simulink model "Simplified_Wind_Turbine_model"  (R2023b)
settings: Solver=ode23t  StartTime=0.0  StopTime=simT  RelTol=1e-3  AbsTol=1e-3
PreLoadFcn:
  | sscv_wind_turbine_input
values from neighbouring files (symbols this model uses):
  actuatorRampRate = 20    [sscv_wind_turbine_input.m]
  brakePressure = 100    [sscv_wind_turbine_input.m]
  controllerTimeConstant = 2    [sscv_wind_turbine_input.m]
  cumulativeStressThreshold = 1.5e6    (= 1500000)    [sscv_wind_turbine_input.m]
  generatorEfficiency = 90    [sscv_wind_turbine_input.m]
  iGenerationGain = 1    [sscv_wind_turbine_input.m]
  initialOperationTime = 0    [sscv_wind_turbine_input.m]
  inizialStressThreshold = 500e3    (= 500000)    [sscv_wind_turbine_input.m]
  maxPitchAngle = max(pitch)    [sscv_wind_turbine_input.m]
  minPitchAngle = min(pitch)    [sscv_wind_turbine_input.m]
  pGenerationGain = 0.1    [sscv_wind_turbine_input.m]
  pGeneratorBrakeLimit = 0.50    (= 0.5)    [sscv_wind_turbine_input.m]
  pitchBrakeAngle = 95    [sscv_wind_turbine_input.m]
  stressRateRelease = 0.05    [sscv_wind_turbine_input.m]
  transformerRatedPower = 1.8    [sscv_wind_turbine_input.m]
  turbineRatedPower = 1.5    [sscv_wind_turbine_input.m]
  vWindRated = 12    [sscv_wind_turbine_input.m]
  wAtGeneratorRatedPower = wTurbineCutOut*gearRatio    (= 1227.93)    [sscv_wind_turbine_input.m]
  wearRate = 0.033    [sscv_wind_turbine_input.m]
  wGeneratorBrakeLimit = 0.50    (= 0.5)    [sscv_wind_turbine_input.m]
  wTurbineCutOut = 22    [sscv_wind_turbine_input.m]
undefined symbols (not defined in the file or in its folder): Derating, mpptOmega, mpptPower, mpptWindSpeed
libraries: fl_lib x22, simulink x14, nesl_utility x11, sdl_lib x10, dspnetwork x3, simulink_extras x3
(part 2 of 2)

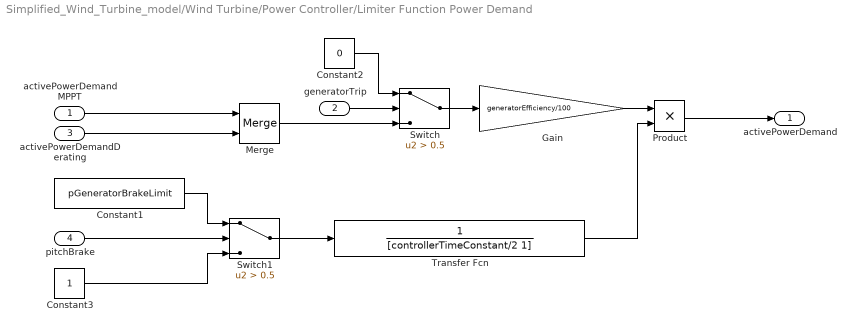
== system Simplified_Wind_Turbine_model/Wind Turbine/Power Controller/Limiter Function Power Demand ==
  activePowerDemandMPPT : Inport
  generatorTrip : Inport  Port=2
  activePowerDemandDerating : Inport  Port=3
  pitchBrake : Inport  Port=4
  Constant1 : Constant  Value=pGeneratorBrakeLimit
  Constant2 : Constant  Value=0
  Constant3 : Constant
  Gain : Gain  Gain=generatorEfficiency/100
  Merge : Merge
  Product : Product
  Switch : Switch  Criteria=u2 > Threshold  Threshold=0.5  SaturateOnIntegerOverflow=off  InputSameDT=off
  Switch1 : Switch  Criteria=u2 > Threshold  Threshold=0.5  SaturateOnIntegerOverflow=off  InputSameDT=off
  Transfer Fcn : TransferFcn  Denominator=[controllerTimeConstant/2 1]
  activePowerDemand : Outport
  wires:
  generatorTrip/1 -> Switch/2
  Switch/1 -> Gain/1
  Constant2/1 -> Switch/1
  Merge/1 -> Switch/3
  activePowerDemandMPPT/1 -> Merge/1
  activePowerDemandDerating/1 -> Merge/2
  pitchBrake/1 -> Switch1/2
  Constant3/1 -> Switch1/3
  Constant1/1 -> Switch1/1
  Gain/1 -> Product/1
  Switch1/1 -> Transfer Fcn/1
  Product/1 -> activePowerDemand/1
  Transfer Fcn/1 -> Product/2

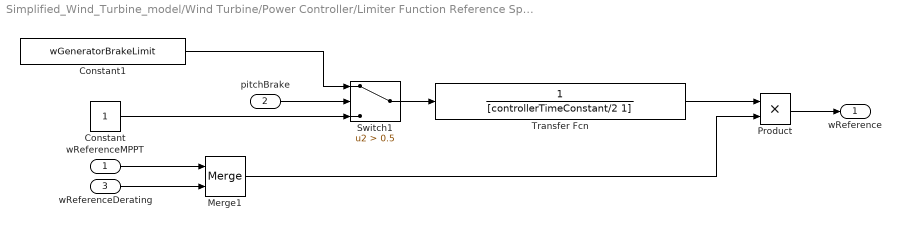
== system Simplified_Wind_Turbine_model/Wind Turbine/Power Controller/Limiter Function Reference Speed ==
  wReferenceMPPT : Inport
  pitchBrake : Inport  Port=2
  wReferenceDerating : Inport  Port=3
  Constant : Constant
  Constant1 : Constant  Value=wGeneratorBrakeLimit
  Merge1 : Merge
  Product : Product
  Switch1 : Switch  Criteria=u2 > Threshold  Threshold=0.5  SaturateOnIntegerOverflow=off  InputSameDT=off
  Transfer Fcn : TransferFcn  Denominator=[controllerTimeConstant/2 1]
  wReference : Outport
  wires:
  pitchBrake/1 -> Switch1/2
  Constant1/1 -> Switch1/1
  wReferenceMPPT/1 -> Merge1/1
  wReferenceDerating/1 -> Merge1/2
  Merge1/1 -> Product/2
  Constant/1 -> Switch1/3
  Product/1 -> wReference/1
  Transfer Fcn/1 -> Product/1
  Switch1/1 -> Transfer Fcn/1

== system Simplified_Wind_Turbine_model/Wind Turbine/Power Controller/MPPT Control ==
  windSpeed : Inport
  Enable : EnablePort  StatesWhenEnabling=reset
  MW to W : Gain  Gain=1e6
  mpptActivePowerDemand : Lookup_n-D  NumberOfTableDimensions=1  BreakpointsForDimension1=mpptWindSpeed  BeginIndexSearchUsingPreviousIndexResult=on  Table=mpptPower  InternalRulePriority=Speed  RndMeth=Simplest
  mpptOmega : Lookup_n-D  NumberOfTableDimensions=1  BreakpointsForDimension1=mpptWindSpeed  BeginIndexSearchUsingPreviousIndexResult=on  Table=mpptOmega  InternalRulePriority=Speed  RndMeth=Simplest
  wReference : Outport
  activePowerDemand : Outport  Port=2
  wires:
  mpptActivePowerDemand/1 -> MW to W/1
  mpptOmega/1 -> wReference/1
  windSpeed/1 -> mpptActivePowerDemand/1, mpptOmega/1
  MW to W/1 -> activePowerDemand/1

== system Simplified_Wind_Turbine_model/Wind Turbine/Gear Tain/Overstress Detector/FaultSystem ==
  Stress : Inport
  StressThreshold : Inport  Port=2
  Compare To Constant : simulink/Logic and Bit Operations/Compare To Constant  relop=>  const=cumulativeStressThreshold  OutDataTypeStr=boolean
  Gain : Gain  Gain=-1*stressRateRelease
  Integrator : Integrator
  Relational Operator : RelationalOperator  Operator=>  OutDataTypeStr=boolean  RndMeth=Simplest  InputSameDT=off
  Switch : Switch  Criteria=u2 > Threshold  SaturateOnIntegerOverflow=off  InputSameDT=off
  fault : Outport
  wires:
  Relational Operator/1 -> Switch/2
  Gain/1 -> Switch/3
  Switch/1 -> Integrator/1
  Integrator/1 -> Compare To Constant/1, Gain/1  "Cumulative Stress"
  StressThreshold/1 -> Relational Operator/2
  Compare To Constant/1 -> fault/1
  Stress/1 -> Switch/1, Relational Operator/1

== system Simplified_Wind_Turbine_model/Wind Turbine/Gear Tain/Overstress Detector/Wear ==
  Bias : Bias  Bias=initialOperationTime  SaturateOnIntegerOverflow=off
  Constant1 : Constant  Value=1/(365*24*60*60)
  Gain1 : Gain  Gain=-1*wearRate
  Integrator1 : Integrator
  Math Function : Math
  Out1 : Outport
  wires:
  Gain1/1 -> Math Function/1
  Constant1/1 -> Integrator1/1
  Math Function/1 -> Out1/1
  Integrator1/1 -> Bias/1
  Bias/1 -> Gain1/1

== stateflow chart Simplified_Wind_Turbine_model/Turbine State Machine ==
  state Startup
    entry: parkingBrake = 0;
    generatorTrip = 1;
    pitchBrake = 0;
    turbineState = 1;
  state Generating
    entry: parkingBrake = 0;
    generatorTrip = 0;
    pitchBrake = 0;
    turbineState = 2;
  state ParkBrake
    entry: parkingBrake = 1;
    generatorTrip = 1;
    pitchBrake = 1;
    turbineState = 0;
  state PitchBrake
    entry: parkingBrake = 0;
    generatorTrip = 0;
    pitchBrake = 1;
    turbineState = 3;
  (junction 37) -> Startup : [duration(windSpeed>...
      | wind_speed_cut_in_lower)>0.10...
      | &&duration(windSpeed<...
      | wind_speed_cut_out)>0.10]
  ParkBrake -> (junction 37)
  Startup -> (junction 41) [order 1] : [duration(turbineSpeed>...
      | turbine_speed_cut_in)>0.10]
  (junction 41) -> Generating
  Startup -> PitchBrake [order 2] : [duration(windSpeed<...
      | wind_speed_cut_in_lower)>1.0...
      | ||duration(windSpeed>...
      | wind_speed_cut_out)>1.0]
  PitchBrake -> Startup [order 2] : [duration(windSpeed<=...
      | wind_speed_cut_in_upper)>2.0...
      | && duration(windSpeed>...
      | wind_speed_cut_in_lower)>2.0...
      | && duration(turbineSpeed<...
      | turbine_speed_cut_in)>2.0]
  (default) -> ParkBrake
  Generating -> (junction 43) : [duration(windSpeed<...
      | wind_speed_cut_in_lower)>0.10...
      | ||duration(windSpeed>...
      | wind_speed_cut_out)>0.10...
      | ||duration(turbineSpeed>...
      | turbine_speed_cut_out)>0.10...
      | ||duration(turbineSpeed<...
      | turbine_speed_cut_in)>0.10]
  (junction 39) -> ParkBrake
  PitchBrake -> (junction 39) [order 1] : [duration(turbineSpeed<=...
      | park_speed)>0.10]
  (junction 43) -> PitchBrake
  data: pitchBrake output double; windSpeed input; turbineSpeed input; parkingBrake output double; generatorTrip output double; wind_speed_cut_in_lower local double =vWindCutInLower; turbine_speed_cut_in local double =wTurbineCutIn; turbineState output double; wind_speed_cut_out local double =vWindCutOut; wind_speed_cut_in_upper local double =vWindCutInUpper; turbine_speed_cut_out local double =wTurbineCutOut; park_speed constant double =wTurbinePark

== matlab function Simplified_Wind_Turbine_model/PLC Connection Interface/Decode data ==
  data: data input; b0 output; b1 output; b2 output
function [b0, b1, b2]= fcn(data)

dec_data = int2bit(data, 3);
b0 = dec_data(1);
b1 = dec_data(2);
b2 = dec_data(3);

== matlab function Simplified_Wind_Turbine_model/PLC Connection Interface/Decode state ==
  data: data input; state output
function state = fcn(data)

if data == 1
    state = 1;
elseif data == 2
    state = 3;
elseif data == 7
    state = 0;
else
    state = 2;
end
